simulink model "ISTrain2025"  (R2025b)
settings: Solver=ode4  StartTime=0.0  StopTime=StopTime  FixedStep=StepSize  RelTol=1e-3
values from neighbouring files (symbols this model uses):
  Crr = 0.004    [MotorScript_ISTrain2025.m]
  G = 10    [MotorScript_ISTrain2025.m]
  g = 9.81    [MotorScript_ISTrain2025.m]
  kc = Simulink.Parameter(0.193);    kc.CoderInfo.StorageClass = 'SimulinkGlobal'    [MotorScript_ISTrain2025.m]
  Ke = Simulink.Parameter(0.138);   Ke.CoderInfo.StorageClass = 'SimulinkGlobal'    [MotorScript_ISTrain2025.m]
  kf = Simulink.Parameter(2.6e-4);    kf.CoderInfo.StorageClass = 'SimulinkGlobal'    [MotorScript_ISTrain2025.m]
  Kt = Simulink.Parameter(0.138);   Kt.CoderInfo.StorageClass = 'SimulinkGlobal'    [MotorScript_ISTrain2025.m]
  m_loco = 600    [MotorScript_ISTrain2025.m]
  mech_eff = 0.85    [MotorScript_ISTrain2025.m]
  n_m = 2    [MotorScript_ISTrain2025.m]
  parameters = struct    [MotorScript_ISTrain2025.m]
  R = Simulink.Parameter(0.14);    R.CoderInfo.StorageClass  = 'SimulinkGlobal'    [MotorScript_ISTrain2025.m]
  rw = 0.100    (= 0.1)    [MotorScript_ISTrain2025.m]
  SF = 30    [MotorScript_ISTrain2025.m]
  StepSize = 0.001    [MotorScript_ISTrain2025.m]
undefined symbols (not defined in the file or in its folder): friction_coeff, grade, m_trail
settings Model: Creator=rafae  LastModifiedBy=Lenovo

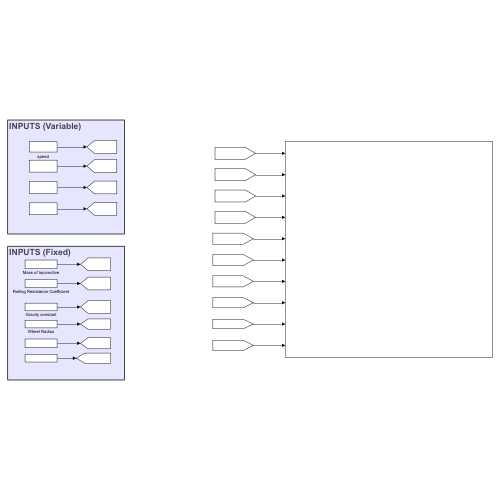
[thumbnail: Simulink's stored preview of the top-level diagram]
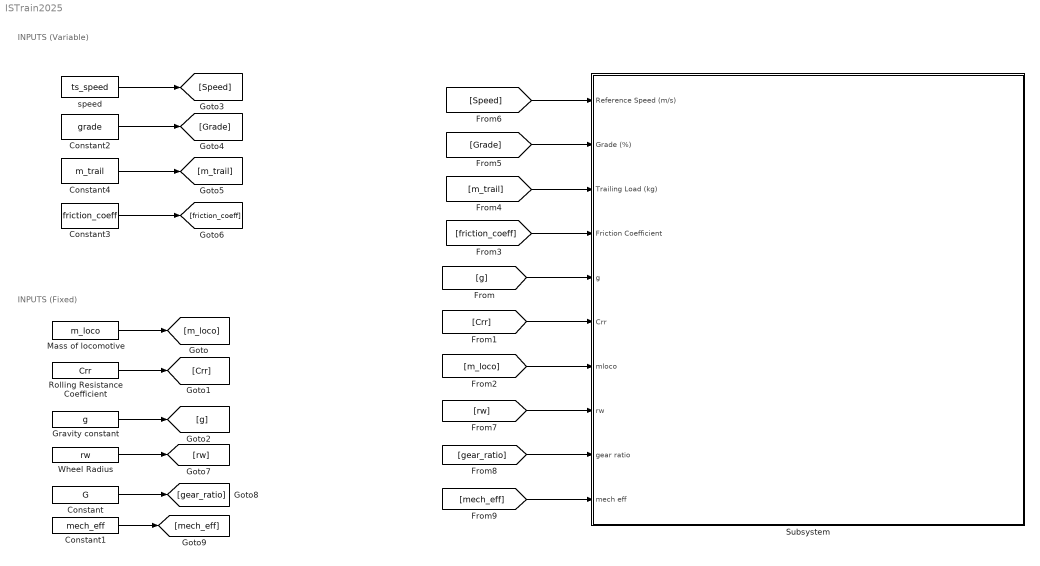
== system ISTrain2025 ==
  note: INPUTS (Variable)
  note: INPUTS (Fixed)
  Constant : Constant  Value=G
  Constant1 : Constant  Value=mech_eff
  Constant2 : Constant  Value=grade
  Constant3 : Constant  Value=friction_coeff
  Constant4 : Constant  Value=m_trail
  Gravity constant : Constant  Value=g
  Mass of locomotive : Constant  Value=m_loco
  Rolling Resistance Coefficient : Constant  Value=Crr
  Subsystem : Subsystem
      mask Display: image('logo_istrain-01.svg');
  Wheel Radius : Constant  Value=rw
  speed : FromWorkspace  VariableName=ts_speed  OutDataTypeStr=double  SampleTime=-1
  wires:
  Constant2/1 -> [Grade]
  Constant4/1 -> [m_trail]
  Mass of locomotive/1 -> [m_loco]
  Rolling Resistance Coefficient/1 -> [Crr]
  Gravity constant/1 -> [g]
  [g] -> Subsystem/5(g)
  [Crr] -> Subsystem/6(Crr)
  [m_loco] -> Subsystem/7(mloco)
  [friction_coeff] -> Subsystem/4(Friction Coefficient)
  [m_trail] -> Subsystem/3(Trailing Load (kg))
  [Grade] -> Subsystem/2(Grade (%))
  [Speed] -> Subsystem/1(Reference Speed (m/s))
  Wheel Radius/1 -> [rw]
  [rw] -> Subsystem/8(rw)
  Constant/1 -> [gear_ratio]
  [gear_ratio] -> Subsystem/9(gear ratio)
  Constant1/1 -> [mech_eff]
  [mech_eff] -> Subsystem/10(mech eff)
  Constant3/1 -> [friction_coeff]
  speed/1 -> [Speed]

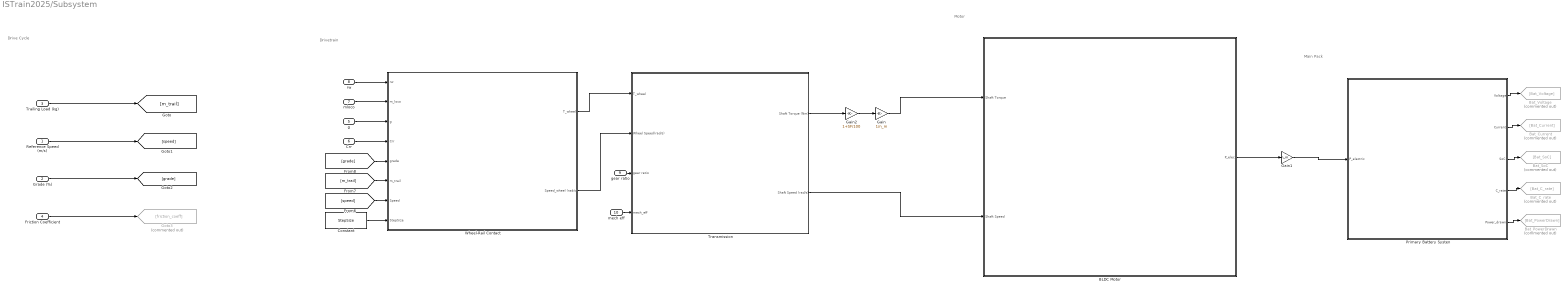
== system ISTrain2025/Subsystem ==
  note: Drive Cycle
  note: Drivetrain
  note: Main Pack
  note: Motor
  Reference Speed (m/s) : Inport
  Grade (%) : Inport  Port=2
  Trailing Load (kg) : Inport  Port=3
  Friction Coefficient : Inport  Port=4
  g : Inport  Port=5
  Crr : Inport  Port=6
  mloco : Inport  Port=7
  rw : Inport  Port=8
  gear ratio : Inport  Port=9
  mech eff : Inport  Port=10
  BLDC Motor : Subsystem
      mask Display: image('Captura de ecrã 2025-11-20 143050.png');
  Bat_C_rate : Goto  Commented=on  GotoTag=Bat_C_rate
  Bat_Current : Goto  Commented=on  GotoTag=Bat_Current
  Bat_PowerDrawn : Goto  Commented=on  GotoTag=Bat_PowerDrawn
  Bat_SoC : Goto  Commented=on  GotoTag=Bat_SoC
  Bat_Voltage : Goto  Commented=on  GotoTag=Bat_Voltage
  Constant : Constant  Value=StepSize
  Gain : Gain  Gain=1/n_m
  Gain1 : Gain  Gain=n_m
  Gain2 : Gain  Gain=1+SF/100
  Goto3 : Goto  Commented=on  GotoTag=friction_coeff
  Primary Battery Systen : Subsystem
      mask Display: image('battery.png');
  Transmission : Subsystem
      mask Display: image('2Q__.jpg');
  Wheel-Rail Contact : Subsystem
      mask Display: image('Rollingstock_axle.jpg');
  wires:
  Primary Battery Systen/1(Voltage) -> Bat_Voltage/1
  Primary Battery Systen/2(Current) -> Bat_Current/1
  Primary Battery Systen/3(SoC) -> Bat_SoC/1
  Primary Battery Systen/5(Power_drawn) -> Bat_PowerDrawn/1
  Primary Battery Systen/4(C_rate) -> Bat_C_rate/1
  Grade (%)/1 -> [grade]
  Trailing Load (kg)/1 -> [m_trail]
  Friction Coefficient/1 -> Goto3/1
  Reference Speed (m/s)/1 -> [speed]
  g/1 -> Wheel-Rail Contact/3(g)
  Crr/1 -> Wheel-Rail Contact/4(Crr)
  mloco/1 -> Wheel-Rail Contact/2(m_loco)
  ? -> ?
  [grade] -> Wheel-Rail Contact/5(grade)
  [m_trail] -> Wheel-Rail Contact/6(m_trail)
  [speed] -> Wheel-Rail Contact/7(Speed)
  rw/1 -> Wheel-Rail Contact/1(rw)
  Wheel-Rail Contact/1(T_wheel) -> Transmission/1(T_wheel)
  Wheel-Rail Contact/2(Speed_wheel (rad/s)) -> Transmission/2(Wheel Speed(rad/s))
  gear ratio/1 -> Transmission/3(gear ratio)
  mech eff/1 -> Transmission/4(mech_eff)
  Transmission/1(Shaft Torque (Nm)) -> Gain2/1
  Transmission/2(Shaft Speed (rad/s)) -> BLDC Motor/2(Shaft Speed)
  Gain/1 -> BLDC Motor/1(Shaft Torque)
  BLDC Motor/1(P_elec) -> Gain1/1
  Gain1/1 -> Primary Battery Systen/1(P_electric)
  Constant/1 -> Wheel-Rail Contact/8(StepSize)
  Gain2/1 -> Gain/1

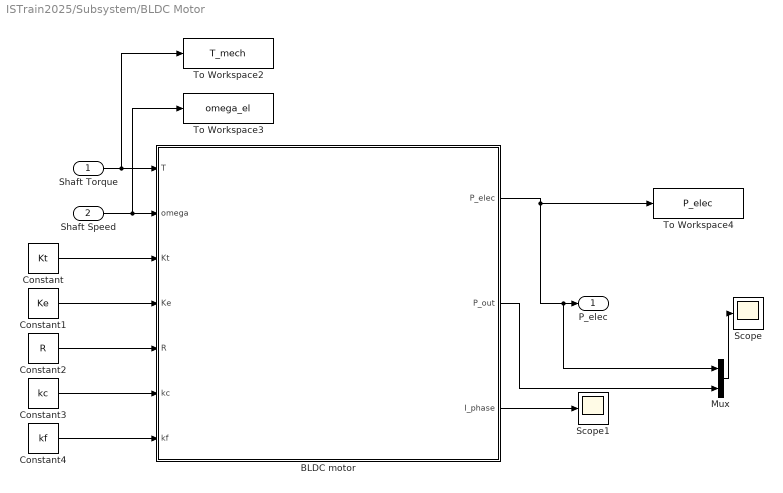
== system ISTrain2025/Subsystem/BLDC Motor ==
  Shaft Torque : Inport
  Shaft Speed : Inport  Port=2
  BLDC motor : MATLAB Function  InitFcn=""  TreatAsAtomicUnit=on
  Constant : Constant  Value=Kt
  Constant1 : Constant  Value=Ke
  Constant2 : Constant  Value=R
  Constant3 : Constant  Value=kc
  Constant4 : Constant  Value=kf
  Mux : Mux  Inputs=2
  Scope : Scope
      settings: ActiveDisplayYMinimum=-6255.3768862692459  ActiveDisplayYMaximum=11488.893381770382  DataLoggingVariableName=ScopeData7
  Scope1 : Scope
      settings: ActiveDisplayYMinimum=-6255.3768862692459  ActiveDisplayYMaximum=11488.893381770382
  To Workspace2 : ToWorkspace  VariableName=T_mech  SaveFormat=Structure With Time  SampleTime=-1
  To Workspace3 : ToWorkspace  VariableName=omega_el  SaveFormat=Structure With Time  SampleTime=-1
  To Workspace4 : ToWorkspace  VariableName=P_elec  SaveFormat=Structure With Time  SampleTime=-1
  P_elec : Outport
  wires:
  Shaft Speed/1 -> To Workspace3/1, BLDC motor/2(omega)
  Shaft Torque/1 -> To Workspace2/1, BLDC motor/1(T)
  BLDC motor/1(P_elec) -> Mux/1, P_elec/1, To Workspace4/1
  Constant/1 -> BLDC motor/3(Kt)
  Constant1/1 -> BLDC motor/4(Ke)
  Constant2/1 -> BLDC motor/5(R)
  Constant3/1 -> BLDC motor/6(kc)
  Constant4/1 -> BLDC motor/7(kf)
  BLDC motor/2(P_out) -> Mux/2
  Mux/1 -> Scope/1
  BLDC motor/3(I_phase) -> Scope1/1

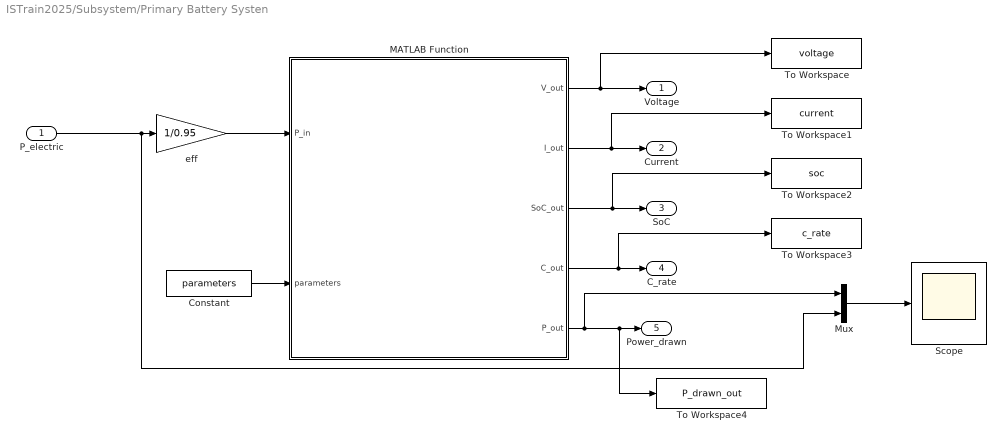
== system ISTrain2025/Subsystem/Primary Battery Systen ==
  P_electric : Inport
  Constant : Constant  Value=parameters  OutDataTypeStr=Bus: parametersBus
  MATLAB Function : MATLAB Function  TreatAsAtomicUnit=on
  Mux : Mux  Inputs=2
  Scope : Scope
      settings: ActiveDisplayYMinimum=-655.81491941325248  ActiveDisplayYMaximum=10259.532215638592  DataLoggingVariableName=ScopeData6
  To Workspace : ToWorkspace  VariableName=voltage  SaveFormat=Structure With Time  SampleTime=-1
  To Workspace1 : ToWorkspace  VariableName=current  SaveFormat=Structure With Time  SampleTime=-1
  To Workspace2 : ToWorkspace  VariableName=soc  SaveFormat=Structure With Time  SampleTime=-1
  To Workspace3 : ToWorkspace  VariableName=c_rate  SaveFormat=Structure With Time  SampleTime=-1
  To Workspace4 : ToWorkspace  VariableName=P_drawn_out  SaveFormat=Structure With Time  SampleTime=-1
  eff : Gain  Gain=1/0.95
  Voltage : Outport
  Current : Outport  Port=2
  SoC : Outport  Port=3
  C_rate : Outport  Port=4
  Power_drawn : Outport  Port=5
  wires:
  MATLAB Function/1(V_out) -> To Workspace/1, Voltage/1
  MATLAB Function/2(I_out) -> To Workspace1/1, Current/1
  MATLAB Function/3(SoC_out) -> To Workspace2/1, SoC/1
  MATLAB Function/4(C_out) -> To Workspace3/1, C_rate/1
  MATLAB Function/5(P_out) -> Mux/1, To Workspace4/1, Power_drawn/1
  Constant/1 -> MATLAB Function/2(parameters)
  eff/1 -> MATLAB Function/1(P_in)
  P_electric/1 -> Mux/2, eff/1
  Mux/1 -> Scope/1

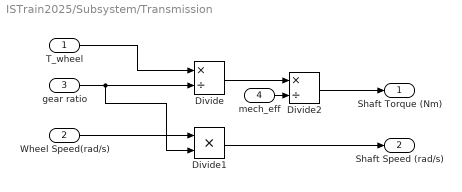
== system ISTrain2025/Subsystem/Transmission ==
  T_wheel : Inport
  Wheel Speed(rad/s) : Inport  Port=2
  gear ratio : Inport  Port=3
  mech_eff : Inport  Port=4
  Divide : Product  Inputs=*/
  Divide1 : Product  Inputs=**
  Divide2 : Product  Inputs=*/
  Shaft Torque (Nm) : Outport
  Shaft Speed (rad/s) : Outport  Port=2
  wires:
  gear ratio/1 -> Divide1/2, Divide/2
  T_wheel/1 -> Divide/1
  Divide/1 -> Divide2/1
  Wheel Speed(rad/s)/1 -> Divide1/1
  Divide1/1 -> Shaft Speed (rad/s)/1
  mech_eff/1 -> Divide2/2
  Divide2/1 -> Shaft Torque (Nm)/1

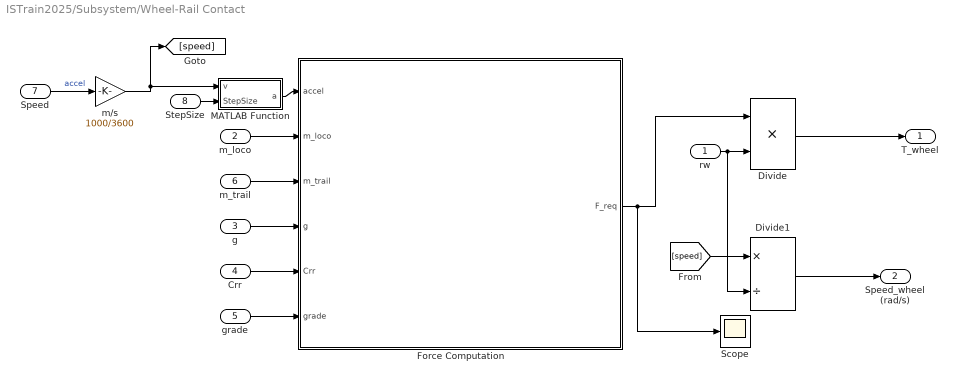
== system ISTrain2025/Subsystem/Wheel-Rail Contact ==
  rw : Inport
  m_loco : Inport  Port=2
  g : Inport  Port=3
  Crr : Inport  Port=4
  grade : Inport  Port=5
  m_trail : Inport  Port=6
  Speed : Inport  Port=7
  StepSize : Inport  Port=8
  Divide : Product  Inputs=**
  Divide1 : Product  Inputs=*/
  Force Computation : MATLAB Function  TreatAsAtomicUnit=on
  MATLAB Function : MATLAB Function  TreatAsAtomicUnit=on
  Scope : Scope
      settings: ActiveDisplayYMinimum=-1  ActiveDisplayYMaximum=1
  m/s : Gain  Gain=1000/3600
  T_wheel : Outport
  Speed_wheel (rad/s) : Outport  Port=2
  wires:
  g/1 -> Force Computation/4(g)
  m_loco/1 -> Force Computation/2(m_loco)
  Crr/1 -> Force Computation/5(Crr)
  grade/1 -> Force Computation/6(grade)
  m_trail/1 -> Force Computation/3(m_trail)
  MATLAB Function/1(a) -> Force Computation/1(accel)
  Speed/1 -> m/s/1  "accel"
  rw/1 -> Divide1/2, Divide/2
  Force Computation/1(F_req) -> Scope/1, Divide/1
  Divide1/1 -> Speed_wheel (rad/s)/1
  [speed] -> Divide1/1
  m/s/1 -> [speed], MATLAB Function/1(v)
  StepSize/1 -> MATLAB Function/2(StepSize)
  Divide/1 -> T_wheel/1

== matlab function ISTrain2025/Subsystem/Primary Battery Systen/MATLAB Function ==
  data: P_in input; V_out output; I_out output; SoC_out output; C_out output; P_out output; parameters input
function [V_out, I_out, SoC_out, C_out, P_out] = batteryModelFcn(P_in, parameters)
%#codegen
persistent SoC V_RC
dt = 0.001;

% Initialize persistent states
if isempty(SoC)
    SoC = 1;           % Start fully charged
end
if isempty(V_RC)
    V_RC = 0;          % RC voltage
end

% Unpack parameters
usable_capacity_Ah = parameters.usable_capacity_Ah;
Q_total            = usable_capacity_Ah * 3600; % [Coulombs]
pack_voltage_nom   = parameters.pack_voltage_nom;
R0                 = parameters.R0;
R1                 = parameters.R1;
C1                 = parameters.C1;
voc_min            = parameters.voc_min;
soc_points         = parameters.soc_points;
voc_points         = parameters.voc_points;
I_max              = parameters.I_max;

% Open-circuit voltage from SoC
Voc = interp1(soc_points, voc_points, SoC, 'linear','extrap');

% If SoC or voltage too low, shut off
if SoC <= 0.1
    I = 0;
    V_terminal = voc_min;
    P_out = 0;
else
    I = P_in / max(Voc, 1e-3);  % Prevent div by zero
end

% Apply current limit
if I > I_max
    I = I_max;
    P_out = I * Voc;
else
    P_out = P_in;
end

% RC branch dynamics
dV_RC = (-V_RC + I * R1) / (R1 * C1) * dt;
V_RC = V_RC + dV_RC;

% Terminal voltage
V_terminal = Voc - I * R0 - V_RC;

% Voltage cutoff
if V_terminal < voc_min
    V_terminal = voc_min;
    I = 0;
    P_out = 0;
end

% Update SoC
dQ = I * dt;
Q_used = (1 - SoC) * Q_total + dQ;
SoC = max(0, 1 - Q_used / Q_total);

% Outputs
V_out   = V_terminal;
I_out   = I;
SoC_out = SoC;
C_out   = I / usable_capacity_Ah;   % C-rate
end

== matlab function ISTrain2025/Subsystem/Wheel-Rail Contact/MATLAB Function ==
  data: v input; a output; StepSize input
function a = diff_accel(v,StepSize)
  % v is the current speed [m/s]
  persistent v_last
  if isempty(v_last)
    v_last = v;
  end
  a = (v - v_last) / StepSize;   % StepSize must be in base workspace
  v_last = v;
end

== matlab function ISTrain2025/Subsystem/Wheel-Rail Contact/Force Computation ==
  data: accel input; m_loco input; m_trail input; F_req output; g input; Crr input; grade input
function F_req = Force_Computation(accel, m_loco, m_trail, g, Crr, grade)

a=accel;
m_total=m_trail+m_loco;

F_grade = m_total * g * grade;  % grade
F_rr    = m_total * g * Crr;% rolling
F_a=m_total*a; % Force due to a imposed acceleration
F_req   = F_grade + F_rr+F_a;
end

== matlab function ISTrain2025/Subsystem/BLDC Motor/BLDC motor ==
  data: T input; P_elec output; omega input; Kt input; Ke input; R input; kc input; kf input; P_out output; I_phase output
function [P_elec,P_out, I_phase]  = calc_elec_power(T, omega, Kt,Ke,R,kc,kf)
  %This function calculates the eletrical power needed for a given
  %mechanical power and a given motor

  % INPUTS:
  %T-Shaft Torque (N.m)
  %omega-Shaft speed (rads-1)
  % motor.Kt  – torque constant [Nm/A]
  % motor.Ke  – EMF constant [V·s/rad]
  % motor.R   – phase resistance [Ohm]
  % motor.kc  – core loss coeff (optional)
  % motor.kf  – friction coeff (optional)

  %OUTPUTS:

  %P_elec-Eletrical Power
  %eff-Motor efficiency
  
  % Phase current from torque
  I_phase   = T / Kt;
  
  % Back-EMF
  E = Ke * omega;
  
  
  % Copper losses
  P_cu = 3 * R * I_phase^2;
  
  % Core losses 
  P_core = kc * omega^2;
  
  % Friction/windage 
  P_fm   = kf * omega;
  
  % Electrical input power
  P_elec = T*omega  + P_cu + P_core + P_fm; % Electrical power
  P_out = T*omega;
  %eff= P_elec/P_mech; % Motor efficiency
end
